simulink model "mcb_ipmsm_pos_est_f28379d_host_model"  (R2023b)
settings: Solver=FixedStepDiscrete  StartTime=0.0  StopTime=inf  RelTol=1e-3  EnableMultiTasking=on
values from neighbouring files (symbols this model uses):
  dataType = 'single'    [mcb_ipmsm_pos_est_f28379d_data.m]
  Ts = T_pwm    (= 5e-05)    [mcb_ipmsm_pos_est_f28379d_data.m]
libraries: instrumentseriallib x4, simulink x3
settings Model: Creator=The MathWorks, Inc.  LastModifiedBy=The MathWorks, Inc.
settings SolverCC: AlgebraicLoopSolver=TrustRegion  MaxZcPerStep=1
settings DataIOCC: LimitDataPoints=on  SaveFormat=Array  ReturnWorkspaceOutputs=off
settings OptimizationCC: ReuseModelBlockBuffer=off  LifeSpan=1  EfficientTunableParamExpr=on
settings DebuggingCC: UnderspecifiedInitializationDetection=Classic  MergeDetectMultiDrivingBlocksExec=none  SolverPrmCheckMsg=warning  ParameterPrecisionLossMsg=none  UnconnectedInputMsg=warning  UnconnectedOutputMsg=warning  UnconnectedLineMsg=warning  AllowSymbolicDim=off  PregeneratedLibrarySubsystemCodeDiagnostic=none  SFUnexpectedBacktrackingDiag=warning  SFNoUnconditionalDefaultTransitionDiag=warning  SFExecutionAtInitializationDiag=none  ArithmeticOperatorsInVariantConditions=warning
settings HardwareCC: ProdBitPerPointer=32  ProdLargestAtomicFloat=None  ProdIntDivRoundTo=Undefined  ProdEndianess=Unspecified  ProdWordSize=32  ProdHWDeviceType=32-bit Generic
settings ModelReferenceCC: EnableRefExpFcnMdlSchedulingChecks=on  PropagateSignalLabelsOutOfModel=off
settings SFSimCC: SimUseLocalCustomCode=off  MATLABDynamicMemAlloc=off
settings RTWCC: Description=Real-Time Workshop Embedded Coder  SystemTargetFile=ert.tlc  TemplateMakefile=ert_default_tmf  GenerateReport=on  RTWUseLocalCustomCode=off  IncludeHyperlinkInReport=on  LaunchReport=on  GenerateTraceInfo=on  GenerateTraceReport=on  GenerateTraceReportSl=on  GenerateTraceReportSf=on  GenerateTraceReportEml=on  DLArmComputeVersion=19.05
settings CodeAppCC: IgnoreCustomStorageClasses=off  StateflowObjectComments=on  InternalIdentifier=Classic
settings ERTTargetCC: MultiwordLength=2048  GenerateSampleERTMain=on  ERTCustomFileTemplate=example_file_process.tlc  ConvertIfToSwitch=off  SuppressUnreachableDefaultCases=off
settings ConfigComp: CovMetricSettings=dw  CovSaveCumulativeToWorkspaceVar=on  CovSaveSingleToWorkspaceVar=on  CovExternalEMLEnable=off  CovSFcnEnable=off

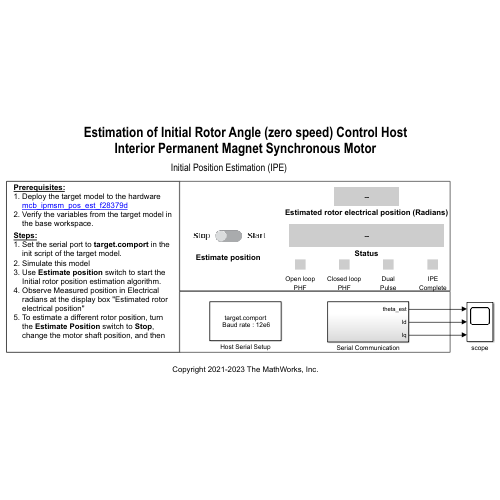
[thumbnail: Simulink's stored preview of the top-level diagram]
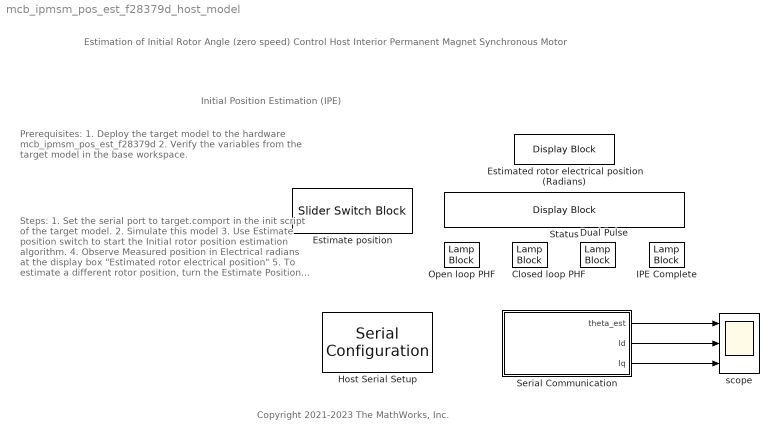
== system mcb_ipmsm_pos_est_f28379d_host_model ==
  note: Estimation of Initial Rotor Angle (zero speed) Control Host
      | Interior Permanent Magnet Synchronous Motor
  note: Copyright 2021-2023 The MathWorks, Inc.
  note: Prerequisites:
      | 1. Deploy the target model to the hardware
      | mcb_ipmsm_pos_est_f28379d
      | 2. Verify the variables from the target model in
      | the base workspace.
  note: Steps:
      | 1. Set the serial port to target.comport in the
      | init script of the target model.
      | 2. Simulate this model
      | 3. Use Estimate position switch to start the
      | Initial rotor position estimation algorithm.
      | 4. Observe Measured position in Electrical
      | radians at the display box "Estimated rotor
      | electrical position"
      | 5. To estimate a different rotor position, turn
      | the Estimate Position switch to Stop ,
      | change the motor shaft position, and then
      | restart the algorithm.
  note: Initial Position Estimation (IPE)
  Closed loop PHF : LampBlock  LabelPosition=Hide  Icon=Square
  Dual Pulse : LampBlock  LabelPosition=Hide  Icon=Square
  "Estimate position " : SliderSwitchBlock  LabelPosition=Hide
      settings: Values={{'Stop', 'Start'}, [0 1]}
  Estimated rotor electrical position (Radians) : DisplayBlock  LabelPosition=Hide  Transparency=1  FormatString=%5d
  Host Serial Setup : instrumentseriallib/Serial Configuration  Priority=-99  PortSel=target.comport  Port=target.comport  ComPort=target.comport  BaudRate=12e6  DataBits=8  Parity=none  StopBits=1  ByteOrder=little-endian  FlowControl=none  Timeout=2  SimulateUsing=Interpreted execution  BlockInModel=on  aMode=5
  IPE Complete : LampBlock  LabelPosition=Hide  Icon=Square
  Open loop PHF : LampBlock  LabelPosition=Hide  Icon=Square
  Serial Communication : Subsystem
  Status : DisplayBlock  LabelPosition=Hide  Transparency=1
  scope : Scope  NumInputPorts=3
  wires:
  Serial Communication/1(theta_est) -> scope/1
  Serial Communication/2(Id) -> scope/2
  Serial Communication/3(Iq) -> scope/3

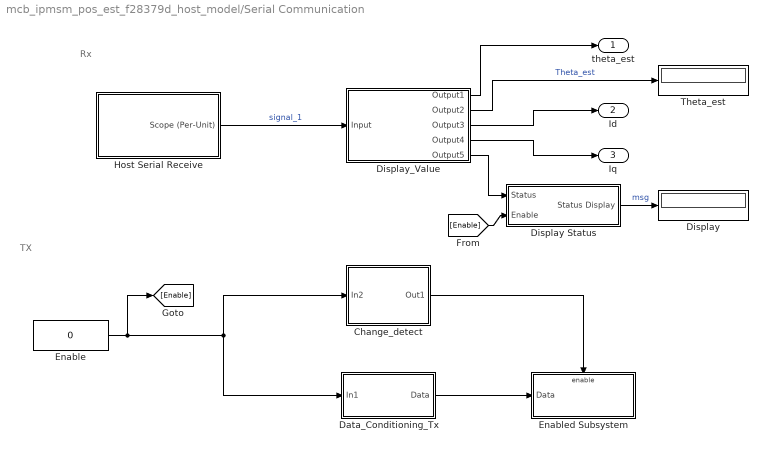
== system mcb_ipmsm_pos_est_f28379d_host_model/Serial Communication ==
  note: TX
  note: Rx
  Change_detect : Subsystem
  Data_Conditioning_Tx : Subsystem  Variant=on
  Display : Display
  Display Status : Subsystem
  Display_Value : MATLAB Function  TreatAsAtomicUnit=on
  Enable : Constant  Value=0  VectorParams1D=off  OutDataTypeStr=uint16  SampleTime=0.03
  Enabled Subsystem : Subsystem  TreatAsAtomicUnit=on
  Host Serial Receive : Subsystem  Variant=on
  Theta_est : Display
  theta_est : Outport
  Id : Outport  Port=2
  Iq : Outport  Port=3
  wires:
  Display_Value/1(Output1) -> theta_est/1
  Host Serial Receive/1(Scope (Per-Unit)) -> Display_Value/1(Input)  "signal_1"
  Enable/1 -> [Enable], Data_Conditioning_Tx/1(In1), Change_detect/1(In2)
  Change_detect/1(Out1) -> Enabled Subsystem/Enable
  Data_Conditioning_Tx/1(Data) -> Enabled Subsystem/1(Data)
  Display_Value/2(Output2) -> Theta_est/1  "Theta_est"
  Display_Value/3(Output3) -> Id/1
  Display_Value/4(Output4) -> Iq/1
  Display_Value/5(Output5) -> Display Status/1(Status)
  Display Status/1(Status Display) -> Display/1  "msg"
  [Enable] -> Display Status/2(Enable)

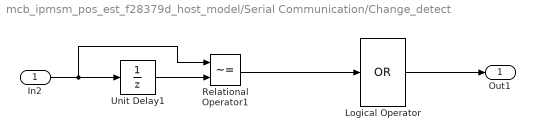
== system mcb_ipmsm_pos_est_f28379d_host_model/Serial Communication/Change_detect ==
  In2 : Inport
  Logical Operator : Logic  Operator=OR  Inputs=1  AllPortsSameDT=off  OutDataTypeStr=boolean
  Relational Operator1 : RelationalOperator  Operator=~=  OutDataTypeStr=boolean  InputSameDT=off
  Unit Delay1 : UnitDelay  SampleTime=-1  HasFrameUpgradeWarning=on
  Out1 : Outport  VectorParamsAs1DForOutWhenUnconnected=off
  wires:
  In2/1 -> Relational Operator1/1, Unit Delay1/1
  Relational Operator1/1 -> Logical Operator/1
  Unit Delay1/1 -> Relational Operator1/2
  Logical Operator/1 -> Out1/1

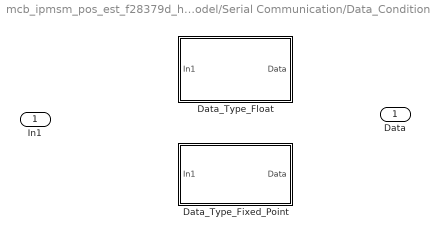
== system mcb_ipmsm_pos_est_f28379d_host_model/Serial Communication/Data_Conditioning_Tx ==
  In1 : Inport
  Data_Type_Fixed_Point : Subsystem  VariantControl=~isequal(dataType, 'single')
  Data_Type_Float : Subsystem  VariantControl=isequal(dataType, 'single')
  Data : Outport

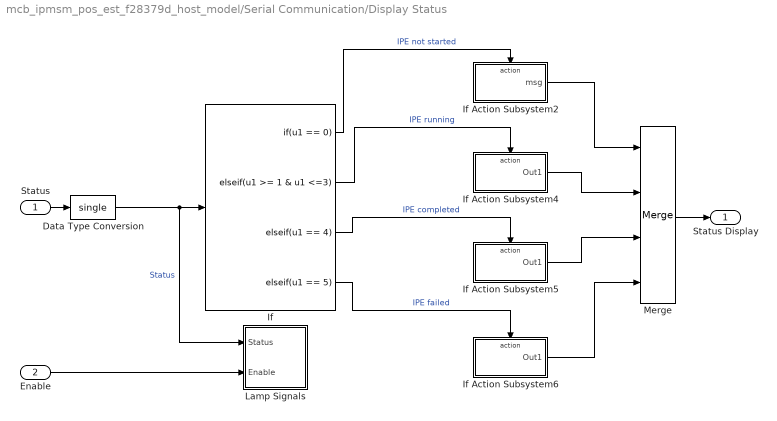
== system mcb_ipmsm_pos_est_f28379d_host_model/Serial Communication/Display Status ==
  Status : Inport
  Enable : Inport  Port=2
  Data Type Conversion : DataTypeConversion  OutDataTypeStr=single  SaturateOnIntegerOverflow=off  RndMeth=Floor
  If : If  IfExpression=u1 == 0  ElseIfExpressions=u1 >= 1 & u1 <=3, u1 == 4, u1 == 5  ShowElse=off
  If Action Subsystem2 : Subsystem  TreatAsAtomicUnit=on
  If Action Subsystem4 : Subsystem  TreatAsAtomicUnit=on
  If Action Subsystem5 : Subsystem  TreatAsAtomicUnit=on
  If Action Subsystem6 : Subsystem  TreatAsAtomicUnit=on
  Lamp Signals : Subsystem
  Merge : Merge  Inputs=4
  Status Display : Outport
  wires:
  Data Type Conversion/1 -> Lamp Signals/1(Status), If/1  "Status"
  If/1 -> If Action Subsystem2/Action  "IPE not started"
  If/3 -> If Action Subsystem5/Action  "IPE completed"
  If/4 -> If Action Subsystem6/Action  "IPE failed"
  Merge/1 -> Status Display/1
  If Action Subsystem2/1(msg) -> Merge/1
  Status/1 -> Data Type Conversion/1
  If/2 -> If Action Subsystem4/Action  "IPE running"
  If Action Subsystem4/1(Out1) -> Merge/2
  If Action Subsystem5/1(Out1) -> Merge/3
  If Action Subsystem6/1(Out1) -> Merge/4
  Enable/1 -> Lamp Signals/2(Enable)

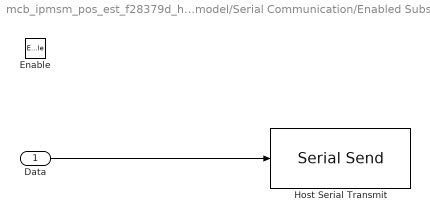
== system mcb_ipmsm_pos_est_f28379d_host_model/Serial Communication/Enabled Subsystem ==
  Data : Inport
  Enable : EnablePort
  Host Serial Transmit : instrumentseriallib/Serial Send  PortSel=target.comport  Port=target.comport  ComPort=target.comport  Header=[]  Terminator=<none>  CustomTerminator=[]  EnableBlockingMode=off  SimulateUsing=Interpreted execution  BlockInModel=on  aMode=5
  wires:
  Data/1 -> Host Serial Transmit/1

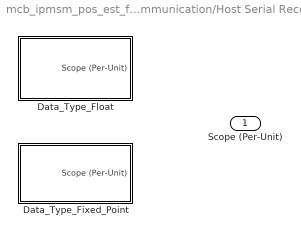
== system mcb_ipmsm_pos_est_f28379d_host_model/Serial Communication/Host Serial Receive ==
  Data_Type_Fixed_Point : Subsystem  VariantControl=~isequal(dataType, 'single')
  Data_Type_Float : Subsystem  VariantControl=isequal(dataType, 'single')
  Scope (Per-Unit) : Outport

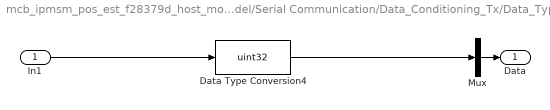
== system mcb_ipmsm_pos_est_f28379d_host_model/Serial Communication/Data_Conditioning_Tx/Data_Type_Fixed_Point ==
  In1 : Inport
  Data Type Conversion4 : DataTypeConversion  OutDataTypeStr=uint32  RndMeth=Simplest  SaturateOnIntegerOverflow=off
  Mux : Mux  Inputs=1
  Data : Outport
  wires:
  Mux/1 -> Data/1
  In1/1 -> Data Type Conversion4/1
  Data Type Conversion4/1 -> Mux/1

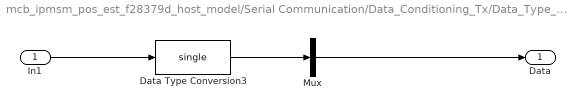
== system mcb_ipmsm_pos_est_f28379d_host_model/Serial Communication/Data_Conditioning_Tx/Data_Type_Float ==
  In1 : Inport
  Data Type Conversion3 : DataTypeConversion  OutDataTypeStr=single  RndMeth=Simplest  SaturateOnIntegerOverflow=off
  Mux : Mux  Inputs=1
  Data : Outport
  wires:
  Mux/1 -> Data/1
  In1/1 -> Data Type Conversion3/1
  Data Type Conversion3/1 -> Mux/1

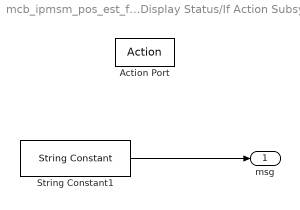
== system mcb_ipmsm_pos_est_f28379d_host_model/Serial Communication/Display Status/If Action Subsystem2 ==
  Action Port : ActionPort  ActionPortLabel=if(u1 == 0)
  String Constant1 : StringConstant  String="\"IPE not started\""
  msg : Outport
  wires:
  String Constant1/1 -> msg/1

== system mcb_ipmsm_pos_est_f28379d_host_model/Serial Communication/Display Status/If Action Subsystem4 ==
  Action Port : ActionPort  ActionPortLabel=elseif(u1 >= 1 & u1 <=3)
  String Constant1 : StringConstant  String="\"IPE running\""
  Out1 : Outport
  wires:
  String Constant1/1 -> Out1/1

== system mcb_ipmsm_pos_est_f28379d_host_model/Serial Communication/Display Status/If Action Subsystem5 ==
  Action Port : ActionPort  ActionPortLabel=elseif( u1 == 4)
  String Constant1 : StringConstant  String="\"IPE completed\""
  Out1 : Outport
  wires:
  String Constant1/1 -> Out1/1

== system mcb_ipmsm_pos_est_f28379d_host_model/Serial Communication/Display Status/If Action Subsystem6 ==
  Action Port : ActionPort  ActionPortLabel=elseif( u1 == 5)
  String Constant1 : StringConstant  String="\"IPE failed\""
  Out1 : Outport
  wires:
  String Constant1/1 -> Out1/1

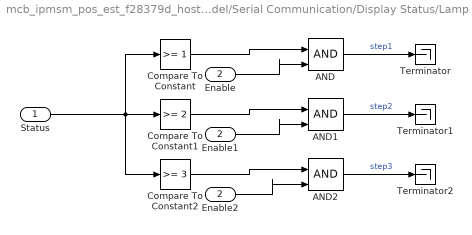
== system mcb_ipmsm_pos_est_f28379d_host_model/Serial Communication/Display Status/Lamp Signals ==
  Status : Inport
  Enable : Inport  Port=2
  AND : Logic  IconShape=distinctive  AllPortsSameDT=off  OutDataTypeStr=boolean
  AND1 : Logic  IconShape=distinctive  AllPortsSameDT=off  OutDataTypeStr=boolean
  AND2 : Logic  IconShape=distinctive  AllPortsSameDT=off  OutDataTypeStr=boolean
  Compare To Constant : simulink/Logic and Bit Operations/Compare To Constant  relop=>=  const=1  OutDataTypeStr=boolean
  Compare To Constant1 : simulink/Logic and Bit Operations/Compare To Constant  relop=>=  const=2  OutDataTypeStr=boolean
  Compare To Constant2 : simulink/Logic and Bit Operations/Compare To Constant  relop=>=  const=3  OutDataTypeStr=boolean
  Enable1 : InportShadow  Port=2
  Enable2 : InportShadow  Port=2
  Terminator : Terminator
  Terminator1 : Terminator
  Terminator2 : Terminator
  wires:
  Status/1 -> Compare To Constant2/1, Compare To Constant/1, Compare To Constant1/1
  AND/1 -> Terminator/1  "step1"
  AND1/1 -> Terminator1/1  "step2"
  AND2/1 -> Terminator2/1  "step3"
  Compare To Constant2/1 -> AND2/1
  Enable2/1 -> AND2/2
  Compare To Constant1/1 -> AND1/1
  Enable1/1 -> AND1/2
  Compare To Constant/1 -> AND/1
  Enable/1 -> AND/2

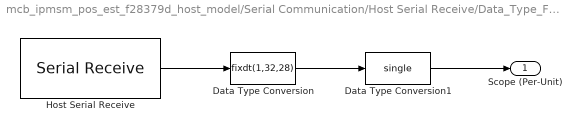
== system mcb_ipmsm_pos_est_f28379d_host_model/Serial Communication/Host Serial Receive/Data_Type_Fixed_Point ==
  Data Type Conversion : DataTypeConversion  OutDataTypeStr=fixdt(1,32,28)  ConvertRealWorld=Stored Integer (SI)  RndMeth=Simplest  SaturateOnIntegerOverflow=off
  Data Type Conversion1 : DataTypeConversion  OutDataTypeStr=single  RndMeth=Simplest  SaturateOnIntegerOverflow=off
  Host Serial Receive : instrumentseriallib/Serial Receive  PortSel=target.comport  Port=target.comport  ComPort=target.comport  DataType=uint32  SaveDataType=uint8  ToggleHeader=on  Header='SSSS'  ToggleTerminator=on  Terminator=Custom terminator  CustomTerminator='EEEE'  InputFormat=Row major  ToggleDataSize=on  DataSize=[600 4]  EnableBlockingMode=on  ActionDataUnavailable=Output custom value  ActionWhenDataUnavailable=Output custom value  CustomValue=10  SampleTime=600*Ts  SimulateUsing=Interpreted execution  BlockInModel=on  aMode=5
  Scope (Per-Unit) : Outport
  wires:
  Data Type Conversion/1 -> Data Type Conversion1/1
  Host Serial Receive/1 -> Data Type Conversion/1
  Data Type Conversion1/1 -> Scope (Per-Unit)/1

== system mcb_ipmsm_pos_est_f28379d_host_model/Serial Communication/Host Serial Receive/Data_Type_Float ==
  Host Serial Receive : instrumentseriallib/Serial Receive  PortSel=target.comport  Port=target.comport  ComPort=target.comport  DataType=single  SaveDataType=uint8  ToggleHeader=on  Header='SSSS'  ToggleTerminator=on  Terminator=Custom terminator  CustomTerminator='EEEE'  InputFormat=Row major  ToggleDataSize=on  DataSize=[600 4]  EnableBlockingMode=on  ActionDataUnavailable=Output custom value  ActionWhenDataUnavailable=Output custom value  CustomValue=10  SampleTime=600*Ts  SimulateUsing=Interpreted execution  BlockInModel=on  aMode=5
  Scope (Per-Unit) : Outport
  wires:
  Host Serial Receive/1 -> Scope (Per-Unit)/1

== matlab function mcb_ipmsm_pos_est_f28379d_host_model/Serial Communication/Display_Value ==
  data: Output1 output; Output2 output; Input input; Output3 output; Output4 output; Output5 output
function [Output1, Output2, Output3, Output4, Output5] = unBuf(Input)

Output1=Input(:,1);
Output2=Output1(1,1);
Output3=Input(:,2);
Output4=Input(:,3);
Status=Input(:,4);
Output5=Status(1,1);

end
